simulink model "atrias_system"  (R2014b)
settings: Solver=FixedStepDiscrete  StartTime=0.0  StopTime=inf  FixedStep=sample_time  RelTol=1e-3
values from neighbouring files (symbols this model uses):
  MEDULLA_TIMER_FREQ = 32e6    (= 32000000)    [Encoder.m]
  sample_time = 0.001    [Encoder.m]
undefined symbols (not defined in the file or in its folder): A_lpf_velocity, B1_lpf_velocity, B2_lpf_velocity, BOOM_MAX_ENCODER_TICKS, BOOM_PITCH_CAL_VALUE_RAD, BOOM_PITCH_CAL_VALUE_TICKS, BOOM_PITCH_ENCODER_RAD_PER_TICK, BOOM_ROLL_CAL_VALUE_RAD, BOOM_ROLL_CAL_VALUE_TICKS, BOOM_ROLL_ENCODER_RAD_PER_TICK, BOOM_YAW_ENCODER_RAD_PER_TICK, fcut_smooth, fcut_unwrap, gui_disable_cmd, gui_enable_cmd, gui_estop_cmd, gui_reset_cmd, HIP_ABS_MAX_ENCODER_TICKS, HIP_CURRENT_LIMIT, HIP_INC_MAX_ENCODER_TICKS, HIP_MOTOR_CONSTANT, HIP_MTR_GEAR_RATIO, HIP_MTR_MAX_TORQUE, isOsuRobot, LEFT_HIP_ABS_ENCODER_RAD_PER_TICK, LEFT_HIP_CALIB_POS, LEFT_HIP_CALIB_VAL, LEFT_HIP_INC_ENCODER_RAD_PER_TICK, LEFT_MOTOR_HIP_DIRECTION, LEG1_LEG_A_CALIB_VAL, LEG1_LEG_A_RAD_PER_CNT, LEG1_LEG_B_CALIB_VAL, LEG1_LEG_B_RAD_PER_CNT, LEG1_MOTOR_A_DIRECTION, LEG1_MOTOR_B_DIRECTION, LEG1_TRAN_A_CALIB_VAL, LEG1_TRAN_A_RAD_PER_CNT, LEG1_TRAN_B_CALIB_VAL, LEG1_TRAN_B_RAD_PER_CNT, LEG2_LEG_A_CALIB_VAL, LEG2_LEG_A_RAD_PER_CNT, LEG2_LEG_B_CALIB_VAL, LEG2_LEG_B_RAD_PER_CNT, LEG2_MOTOR_A_DIRECTION, LEG2_MOTOR_B_DIRECTION, LEG2_TRAN_A_CALIB_VAL, LEG2_TRAN_A_RAD_PER_CNT, LEG2_TRAN_B_CALIB_VAL, LEG2_TRAN_B_RAD_PER_CNT, LEG_A_CALIB_LOC, LEG_B_CALIB_LOC, LEG_CURRENT_LIMIT, LEG_INC_ENCODER_RAD_PER_TICK, LEG_MOTOR_CONSTANT, LEG_MTR_GEAR_RATIO, LEG_MTR_MAX_TORQUE, max_encoder_velocity, max_sensor_velocity, MEDULLA_ADC_MAX_VOLTS, MEDULLA_ADC_OFFSET_COUNTS ... (+17)
libraries: xpcethercatlib x201, simulink x53, slrtlib x2
(part 1 of 4)
settings Model: xpc_rtwmakecfg_data=_xpcethercatlib_  SimulationMode=external  BufferReuse=off  Creator=wmartin  LastModifiedBy=drl
settings SolverCC: EnableConcurrentExecution=on
settings DataIOCC: MaxDataPoints=1000000000  SaveFormat=StructureWithTime  SaveOutput=off  SaveTime=off
settings OptimizationCC: BlockReduction=off  OptimizeBlockIOStorage=off  BufferReuse=off  GlobalBufferReuse=off  ExpressionFolding=off  ExpressionDepthLimit=2147483647  LocalBlockOutputs=off  SimCompilerOptimization=On
settings DebuggingCC: UnderspecifiedInitializationDetection=Classic  MergeDetectMultiDrivingBlocksExec=none  StateNameClashWarn=warning
settings HardwareCC: ProdIntDivRoundTo=Zero  ProdEndianess=LittleEndian  ProdLongLongMode=on  ProdHWDeviceType=Generic->32-bit x86 compatible
settings ModelReferenceCC: EnableParallelModelReferenceBuilds=on  ModelReferenceNumInstancesAllowed=Single  ModelReferenceMinAlgLoopOccurrences=on
settings RTWCC: SystemTargetFile=slrt.tlc  TemplateMakefile=slrt_default_tmf  Description=Simulink Real-Time  RTWVerbose=off  ProcessScript=slrt_make_rtw_hook  RTWCompilerOptimization=On
settings CodeAppCC: MaxIdLength=256
settings SimulinkRealTimeCC: GeneratePreprocessorConditionals=Disable all  EnableShiftOperators=on  RL32LogBufSizeModifier=100000000

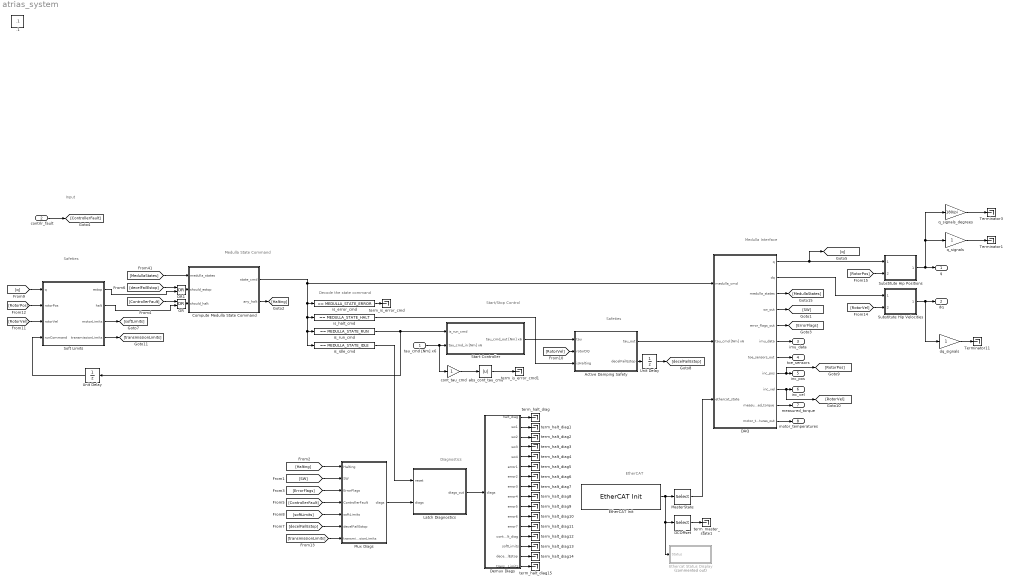
== system atrias_system ==
  note: Decode the state command
  note: Medulla Interface
  note: Medulla State Command
  note: Diagnostics
  note: EtherCAT
  note: Start/Stop Control
  note: Input
  note: Safeties
  note: Safeties
  tau_cmd [Nm] x6 : Inport
  contrlr_fault : Inport  Port=2  OutDataTypeStr=boolean
  Active Damping Safety : MATLAB Function  TreatAsAtomicUnit=on
  Compute Medulla State Command : MATLAB Function  TreatAsAtomicUnit=on
  DAQ : Subsystem
  DCOffset : Selector  InputPortWidth=6  Indices=[4]
  Demux Diags : MATLAB Function  TreatAsAtomicUnit=on
  EtherCAT Init : xpcethercatlib/EtherCAT Init   Priority=0  config_file=8medullas4elmos_eni.xml  device_id=0  pci_bus=2  pci_slot=0  enaDebug=off  enaDC=on  errLink=off  masterDbg=off  stateChgDbg=off  baseClock=off  masterCfg=off  logFile='E:\dbglog.txt'  sample_time=0.001000
  Ethercat Status Display : Subsystem  Commented=on
  Latch Diagnostics : MATLAB Function  TreatAsAtomicUnit=on
  MasterState : Selector  InputPortWidth=6  Indices=[2]
  Mux Diags : MATLAB Function  TreatAsAtomicUnit=on
  OR : Logic  Operator=OR  AllPortsSameDT=off  OutDataTypeStr=boolean
  OR1 : Logic  Operator=OR  AllPortsSameDT=off  OutDataTypeStr=boolean
  Soft Limits : MATLAB Function  TreatAsAtomicUnit=on
  Start Controller : Subsystem
  Substitute Hip Positions : Subsystem
  Substitute Hip Velocities : Subsystem
  Terminator1 : Terminator
  Terminator11 : Terminator
  Terminator3 : Terminator
  Unit Delay : UnitDelay  SampleTime=-1
  "Unit Delay " : UnitDelay  SampleTime=-1
  abs_cont_tau_cmd : Abs
  cont_tau_cmd : Gain
  dq_signals : Gain
  is_error_cmd : simulink/Logic and Bit Operations/Compare To Constant  relop===  const=MEDULLA_STATE_ERROR  OutDataTypeStr=boolean
  is_halt_cmd : simulink/Logic and Bit Operations/Compare To Constant  relop===  const=MEDULLA_STATE_HALT  OutDataTypeStr=boolean
  is_idle_cmd : simulink/Logic and Bit Operations/Compare To Constant  relop===  const=MEDULLA_STATE_IDLE  OutDataTypeStr=boolean
  is_run_cmd : simulink/Logic and Bit Operations/Compare To Constant  relop===  const=MEDULLA_STATE_RUN  OutDataTypeStr=boolean
  q_signals : Gain
  q_signals_degrees : Gain  Gain=180/pi
  term_halt_diag{,1..15} (16 alike) : Terminator
  term_is_error_cmd : Terminator
  term_is_error_cmd1 : Terminator
  term_master_state1 : Terminator
  q : Outport
  dq : Outport  Port=2
  imu_data : Outport  Port=3
  toe_sensors : Outport  Port=4
  inc_pos : Outport  Port=5
  inc_vel : Outport  Port=6
  measured_torque : Outport  Port=7
  motor_temperatures : Outport  Port=8
  .1 : Constant  IOType=siggen  Value=.1
  wires:
  MasterState/1 -> DAQ/3(ethercat_state)
  [MedullaStates] -> Compute Medulla State Command/1(medulla_states)
  Compute Medulla State Command/2(any_halt) -> [Halting]
  Latch Diagnostics/1(diags_out) -> Demux Diags/1(diags)
  is_halt_cmd/1 -> Active Damping Safety/3(isHalting)
  is_error_cmd/1 -> term_is_error_cmd/1
  tau_cmd [Nm] x6/1 -> cont_tau_cmd/1, Start Controller/2(tau_cmd_in [Nm] x6)
  Start Controller/1(tau_cmd_out [Nm] x6) -> Active Damping Safety/1(tau)
  is_idle_cmd/1 -> Latch Diagnostics/1(reset)
  DAQ/4(sw_out) -> [SW]
  Mux Diags/1(diags) -> Latch Diagnostics/2(diags)
  [Halting] -> Mux Diags/1(Halting)
  [SW] -> Mux Diags/2(SW)
  Demux Diags/2(sw1) -> term_halt_diag1/1
  Demux Diags/5(sw4) -> term_halt_diag4/1
  Demux Diags/4(sw3) -> term_halt_diag3/1
  Demux Diags/3(sw2) -> term_halt_diag2/1
  DAQ/5(error_flags_out) -> [ErrorFlags]
  [ErrorFlags] -> Mux Diags/3(ErrorFlags)
  Demux Diags/1(halt_diag) -> term_halt_diag/1
  Demux Diags/12(error7) -> term_halt_diag11/1
  Demux Diags/11(error6) -> term_halt_diag10/1
  Demux Diags/10(error5) -> term_halt_diag9/1
  Demux Diags/9(error4) -> term_halt_diag8/1
  Demux Diags/8(error3) -> term_halt_diag7/1
  Demux Diags/7(error2) -> term_halt_diag6/1
  Demux Diags/6(error1) -> term_halt_diag5/1
  abs_cont_tau_cmd/1 -> term_is_error_cmd1/1
  DAQ/6(imu_data) -> imu_data/1
  [ControllerFault] -> Mux Diags/4(ControllerFault)
  Demux Diags/13(contrlr_fault_diag) -> term_halt_diag12/1
  [RotorPos] -> Soft Limits/2(rotorPos)
  [RotorVel] -> Soft Limits/3(rotorVel)
  EtherCAT Init/1 -> DCOffset/1, Ethercat Status Display/1(Status), MasterState/1
  Compute Medulla State Command/1(state_cmd) -> is_idle_cmd/1, is_run_cmd/1, is_halt_cmd/1, is_error_cmd/1, DAQ/1(medulla_cmd)
  cont_tau_cmd/1 -> abs_cont_tau_cmd/1
  DAQ/7(toe_sensors_out) -> toe_sensors/1
  contrlr_fault/1 -> [ControllerFault]
  [softLimits] -> Mux Diags/5(softLimits)
  Demux Diags/14(softLimits) -> term_halt_diag13/1
  Soft Limits/3(motorLimits) -> [softLimits]
  is_run_cmd/1 -> Unit Delay/1, Start Controller/1(is_run_cmd)
  Active Damping Safety/1(tau_out) -> DAQ/2(tau_cmd [Nm] x6)
  [RotorVel] -> Active Damping Safety/2(rotorDQ)
  DCOffset/1 -> term_master_state1/1
  [q] -> Soft Limits/1(q)
  [decelFailEstop] -> Mux Diags/6(decelFailEstop)
  Demux Diags/15(decelFailEstop) -> term_halt_diag14/1
  DAQ/3(medulla_states) -> [MedullaStates]
  Active Damping Safety/2(decelFailEstop) -> "Unit Delay "/1
  "Unit Delay "/1 -> [decelFailEstop]
  DAQ/10(measured_torque) -> measured_torque/1
  DAQ/9(inc_vel) -> [RotorVel], inc_vel/1
  DAQ/8(inc_pos) -> [RotorPos], inc_pos/1
  [ControllerFault] -> OR/1
  Soft Limits/2(halt) -> OR/2
  OR/1 -> Compute Medulla State Command/3(should_halt)
  Unit Delay/1 -> Soft Limits/4(runCommand)
  [decelFailEstop] -> OR1/1
  OR1/1 -> Compute Medulla State Command/2(should_estop)
  Soft Limits/1(estop) -> OR1/2
  Soft Limits/4(transmissionLimits) -> [transmissionLimits]
  [transmissionLimits] -> Mux Diags/7(transmissionLimits)
  Demux Diags/16(transmissionLimits) -> term_halt_diag15/1
  DAQ/11(motor_temperatures_out) -> motor_temperatures/1
  [RotorVel] -> Substitute Hip Velocities/2(Incremental)
  DAQ/2(dq) -> Substitute Hip Velocities/1(Absolute)
  DAQ/1(q) -> Substitute Hip Positions/1(Absolute), [q]
  [RotorPos] -> Substitute Hip Positions/2(Incremental)
  q_signals/1 -> Terminator1/1
  q_signals_degrees/1 -> Terminator3/1
  Substitute Hip Positions/1(Substituted) -> q_signals_degrees/1, q_signals/1, q/1
  Substitute Hip Velocities/1(Substituted) -> dq_signals/1, dq/1
  dq_signals/1 -> Terminator11/1

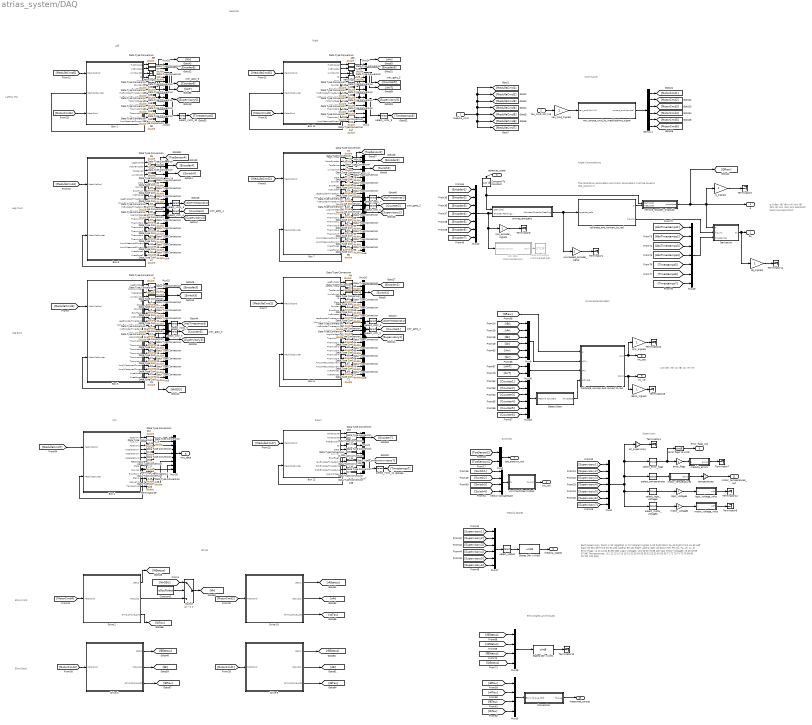
== system atrias_system/DAQ ==
  note: Left
  note: The calibration parameters and motor parameters
      | must be saved in daq_params.m
  note: Right
  note: Lateral Hip
  note: Leg Back
  note: Leg Front
  note: Boom
  note: Medullas
  note: Angle Computations
  note: Commands
  note: Switches
  note: Supervisory
  note: Each Supervisory block is 20 (sagittal) or 12 (lateral) signals
      | 1-20      Right Back
      | 21-40     Right Front
      | 41-60     Left Back
      | 61-80     Left Front
      | 81-92     Left Lateral
      | 93-104    Right Lateral
      | 105-112   Boom
      |
      | BR, FR, BL, FL, LR, LL, B
      | Error Flags: [4 24 44 64 84 96 108]
      | Logic Voltages: [10 30 50 70 88 100 112]
      | Motor Voltages: [9 29 49 69 87 99]
      | Temperatures: [11 12 13 14 15 16 31 32 33 34 35 36 51 52 53 54 55 56 71 72 73 74 75 76 89 90 91 101 102 103]
  note: q Order:
      |
      | rBl
      | rBm
      | rAl
      | rAm
      |
      | lBl
      | lBm
      | lAl
      | lAm
      |
      | rHm
      | lHm
      |
      | boomRoll
      | boomYaw
      | boomPitch
  note: Medulla States
  note: IMU
  note: Elmos
  note: Elmo Front
  note: Elmo Back
  note: Elmo States and Torques
  note: Incremental Encoders
  note: q Order:
      |
      | rBr
      | rAr
      | lBr
      | lAr
      |
      | rHr
      | lHr
  medulla_cmd : Inport
  tau_cmd [Nm] x6 : Inport  Port=2  OutDataTypeStr=double  PortDimensions=6  SampleTime=0
  ethercat_state : Inport  Port=3
  Box 1 : Subsystem
  Box 11 : Subsystem
  Box 12 : Subsystem
  Box 4 : Subsystem
  Box 5 : Subsystem
  Box 6 : Subsystem
  Box 7 : Subsystem
  Box 8 : Subsystem
  "Calibrate, unwrap, and convert to rad" : MATLAB Function  TreatAsAtomicUnit=on
  Compare To Constant : simulink/Logic and Bit Operations/Compare To Constant  relop===  const=8  OutDataTypeStr=boolean
  Constant1 : Constant  Value=isOsuRobot  OutDataTypeStr=Inherit: Inherit via back propagation
  Conversion : Subsystem
  Data Type Conversion{1..120,127..147,149..151} (144 alike) : DataTypeConversion  OutDataTypeStr=double
  Demux1 : Demux  Outputs=6
  Derivative : Subsystem
  Detect Data : Subsystem
  Drive 10 : Subsystem
  Drive 2 : Subsystem
  Drive 3 : Subsystem
  Drive 9 : Subsystem
  Error flags to uint8 : DataTypeConversion  OutDataTypeStr=uint8
  Fail Safe : Subsystem  Commented=on
  Limit Switches to Bool : MATLAB Function  TreatAsAtomicUnit=on
  Mux1 : Mux  Inputs=12
  Mux10 : Mux  Inputs=12
  Mux{2,11..16,18..20,24,30} (12 alike) : Mux  Inputs=2
  Mux17 : Mux  Inputs=6
  Mux21 : Mux  Inputs=3
  Mux22 : Mux  Inputs=7
  Mux23 : Mux  Inputs=6
  Mux25 : Mux
  Mux26 : Mux  Inputs=9
  Mux28 : Mux
  Mux29 : Mux  Inputs=7
  Mux{3..6} (4 alike) : Mux  Inputs=20
  Mux7 : Mux  Inputs=8
  Mux8 : Mux  Inputs=7
  Mux9 : Mux  Inputs=6
  States Dbl->Uint1 : DataTypeConversion  OutDataTypeStr=uint8
  States Dbl->Uint8 : DataTypeConversion  OutDataTypeStr=uint8
  Stop Simulation : Stop  Commented=on
  Switch : Switch  Criteria=u2 ~= 0  Threshold=max_sensor_velocity*sample_time
      settings: AttributesFormatString=%<Criteria>
  Terminator{1,3..4,6..14,19,22..25} (17 alike) : Terminator
  Vector Concatenate : Concatenate  NumInputs=4
  all_supervisory : Gain
  calibrate_and_convert_to_rad : Subsystem
  dq_signals : Gain
  dqinc_signals : Gain
  error_flags : Gain
  logic_voltage_volts : MATLAB Function  TreatAsAtomicUnit=on
  logic_voltages : Gain
  medulla_errors : MATLAB Function  TreatAsAtomicUnit=on
  motor_temperatures : MATLAB Function  TreatAsAtomicUnit=on
  motor_voltage_volts : MATLAB Function  TreatAsAtomicUnit=on
  motor_voltages : Gain
  mtr_torque_cmd_to_medulla/elmo_signal : Subsystem
  q_signals : Gain
  qinc_signals : Gain
  raw_encoder_signals : Gain
  remove_encoder_dropouts : Subsystem
  select_cntr_{1..4} (4 alike) : Selector  InputPortWidth=20  Indices=3
  select_error_flags : Selector  InputPortWidth=112  Indices=[4 24 44 64 84 96 108]
  select_incts_10 : Selector  InputPortWidth=12  Indices=[6]
  select_incts_11 : Selector  InputPortWidth=8  Indices=[5 6 7]
  select_incts_{5..8} (4 alike) : Selector  InputPortWidth=20  Indices=[6 7]
  select_incts_9 : Selector  InputPortWidth=12  Indices=[6]
  select_logic_voltages : Selector  InputPortWidth=112  Indices=[10 30 50 70 88 100 112]
  select_motor_voltages : Selector  InputPortWidth=112  Indices=[9 29 49 69 87 99]
  select_states : Selector  InputPortWidth=104  Indices=[2 22 42 62 82 94]
  select_temperatures : Selector  InputPortWidth=112  Indices=[11 12 13 14 15 16 31 32 33 34 35 36 51 52 53 54 55 56 71 72 73 74 75 76 89 90 91 101 102 103]
  tau_cmd_signals : Gain
  temperatures : Gain
  unwrap_encoders : Subsystem
  unwrapped_encoder_signal : Gain
  q : Outport  OutDataTypeStr=double  PortDimensions=13  SampleTime=[0.001,0]
  dq : Outport  Port=2  OutDataTypeStr=double  PortDimensions=13  SampleTime=[0.001,0]
  medulla_states : Outport  Port=3  OutDataTypeStr=uint8
  sw_out : Outport  Port=4
  error_flags_out : Outport  Port=5  OutDataTypeStr=uint8
  imu_data : Outport  Port=6
  toe_sensors_out : Outport  Port=7
  inc_pos : Outport  Port=8
  inc_vel : Outport  Port=9
  measured_torque : Outport  Port=10
  motor_temperatures_out : Outport  Port=11
  wires:
  Box 12/11(LogicVoltage) -> Data Type Conversion136/1
  Box 12/10(PitchEncoderTimestamp) -> Data Type Conversion137/1
  Box 12/9(RollEncoderTimestamp) -> Data Type Conversion127/1
  Box 12/8(YawEncoderTimestamp) -> Data Type Conversion129/1
  Box 12/7(ErrorFlags) -> Data Type Conversion130/1
  Box 12/5(State) -> Data Type Conversion134/1
  Box 12/4(ID) -> Data Type Conversion135/1
  Box 12/3(PitchEncoder) -> Data Type Conversion131/1
  Box 12/2(YawEncoder) -> Data Type Conversion132/1
  Box 12/1(RollEncoder) -> Data Type Conversion133/1
  Data Type Conversion133/1 -> Mux21/1
  Data Type Conversion132/1 -> Mux21/2
  Data Type Conversion131/1 -> Mux21/3
  Data Type Conversion135/1 -> Mux7/1
  Data Type Conversion134/1 -> Mux7/2
  Data Type Conversion128/1 -> Mux7/3
  Data Type Conversion130/1 -> Mux7/4
  Data Type Conversion129/1 -> Mux7/5
  Data Type Conversion127/1 -> Mux7/6
  Data Type Conversion137/1 -> Mux7/7
  Data Type Conversion136/1 -> Mux7/8
  Data Type Conversion98/1 -> Mux18/1
  Data Type Conversion97/1 -> [lHr], Mux18/2
  Data Type Conversion110/1 -> Mux10/1
  Data Type Conversion105/1 -> Mux10/2
  Data Type Conversion107/1 -> [Counter6], Mux10/3
  Data Type Conversion106/1 -> Mux10/4
  Data Type Conversion109/1 -> Mux10/5
  Data Type Conversion101/1 -> Mux10/7
  Data Type Conversion103/1 -> Mux10/8
  Data Type Conversion102/1 -> Mux10/9
  Data Type Conversion100/1 -> Mux10/10
  Data Type Conversion99/1 -> Mux10/11
  mtr_torque_cmd_to_medulla/elmo_signal/1(current_cmd [counts]) -> Demux1/1
  Data Type Conversion50/1 -> Mux16/2
  Data Type Conversion49/1 -> Mux16/1
  Data Type Conversion48/1 -> Mux4/20
  Data Type Conversion47/1 -> Mux4/19
  Data Type Conversion46/1 -> Mux4/18
  Data Type Conversion45/1 -> Mux4/17
  Data Type Conversion44/1 -> Mux4/16
  Data Type Conversion43/1 -> Mux4/15
  Data Type Conversion42/1 -> Mux4/14
  Data Type Conversion41/1 -> Mux4/13
  Data Type Conversion40/1 -> Mux4/12
  Data Type Conversion39/1 -> Mux4/11
  Data Type Conversion38/1 -> Mux4/10
  Data Type Conversion37/1 -> Mux4/9
  Data Type Conversion36/1 -> Mux4/8
  Data Type Conversion35/1 -> Mux4/7
  Data Type Conversion34/1 -> Mux4/6
  Data Type Conversion33/1 -> Mux4/5
  Data Type Conversion32/1 -> Mux4/4
  Data Type Conversion31/1 -> Mux4/3
  Data Type Conversion30/1 -> Mux4/2
  Data Type Conversion29/1 -> Mux4/1
  Data Type Conversion27/1 -> Mux14/1, [ToeSensor4]
  Data Type Conversion26/1 -> Mux20/2
  Data Type Conversion25/1 -> Mux20/1
  Data Type Conversion24/1 -> Mux3/20
  Data Type Conversion23/1 -> Mux3/19
  Data Type Conversion22/1 -> Mux3/18
  Data Type Conversion21/1 -> Mux3/17
  Data Type Conversion20/1 -> Mux3/16
  Data Type Conversion19/1 -> Mux3/15
  Data Type Conversion18/1 -> Mux3/14
  Data Type Conversion17/1 -> Mux3/13
  Data Type Conversion16/1 -> Mux3/12
  Data Type Conversion15/1 -> Mux3/11
  Data Type Conversion14/1 -> Mux3/10
  Data Type Conversion13/1 -> Mux3/9
  Data Type Conversion12/1 -> Mux3/8
  Data Type Conversion11/1 -> Mux3/7
  Data Type Conversion10/1 -> Mux3/6
  Data Type Conversion9/1 -> [lArOSU], Mux3/5
  Data Type Conversion8/1 -> Mux3/4
  Data Type Conversion7/1 -> Mux3/3
  Data Type Conversion6/1 -> Mux3/2
  Data Type Conversion5/1 -> Mux3/1
  Data Type Conversion2/1 -> Mux13/1
  Data Type Conversion1/1 -> Mux15/2
  Data Type Conversion3/1 -> Mux15/1
  tau_cmd [Nm] x6/1 -> tau_cmd_signals/1
  Data Type Conversion138/1 -> Mux10/12
  Data Type Conversion96/1 -> Mux6/20
  Data Type Conversion95/1 -> Mux6/19
  Data Type Conversion94/1 -> Mux6/18
  Data Type Conversion93/1 -> Mux6/17
  Data Type Conversion92/1 -> Mux6/16
  Data Type Conversion91/1 -> Mux6/15
  Data Type Conversion90/1 -> Mux6/14
  Data Type Conversion89/1 -> Mux6/13
  Data Type Conversion88/1 -> Mux6/12
  Data Type Conversion87/1 -> Mux6/11
  Data Type Conversion86/1 -> Mux6/10
  Data Type Conversion85/1 -> Mux6/9
  Data Type Conversion84/1 -> Mux6/8
  Data Type Conversion83/1 -> Mux6/7
  Data Type Conversion82/1 -> Mux6/6
  Data Type Conversion81/1 -> Mux6/5
  Data Type Conversion80/1 -> Mux6/4
  Data Type Conversion79/1 -> Mux6/3
  Data Type Conversion78/1 -> Mux6/2
  Data Type Conversion77/1 -> Mux6/1
  Data Type Conversion75/1 -> Mux11/1, [ToeSensor2]
  Data Type Conversion74/1 -> Mux19/2
  Data Type Conversion73/1 -> Mux19/1
  Data Type Conversion72/1 -> Mux5/20
  Data Type Conversion71/1 -> Mux5/19
  Data Type Conversion70/1 -> Mux5/18
  Data Type Conversion69/1 -> Mux5/17
  Data Type Conversion68/1 -> Mux5/16
  Data Type Conversion67/1 -> Mux5/15
  Data Type Conversion66/1 -> Mux5/14
  Data Type Conversion65/1 -> Mux5/13
  Data Type Conversion64/1 -> Mux5/12
  Data Type Conversion63/1 -> Mux5/11
  Data Type Conversion62/1 -> Mux5/10
  Data Type Conversion61/1 -> Mux5/9
  Data Type Conversion60/1 -> Mux5/8
  Data Type Conversion59/1 -> Mux5/7
  Data Type Conversion58/1 -> Mux5/6
  Data Type Conversion57/1 -> Mux5/5
  Data Type Conversion56/1 -> Mux5/4
  Data Type Conversion55/1 -> Mux5/3
  Data Type Conversion54/1 -> Mux5/2
  Data Type Conversion53/1 -> Mux5/1
  Data Type Conversion51/1 -> Mux12/1
  Box 12/6(Counter) -> Box 12/2(MedullaCounter), Data Type Conversion128/1
  [MedullaCmd7] -> Box 12/1(MedullaCmd)
  Derivative/1(dq) -> dq_signals/1, dq/1
  Demux1/1 -> [MotorCmd1]
  Demux1/2 -> [MotorCmd2]
  Demux1/3 -> [MotorCmd3]
  Demux1/4 -> [MotorCmd4]
  Demux1/5 -> [MotorCmd5]
  Demux1/6 -> [MotorCmd6]
  Mux3/1 -> select_incts_5/1, select_cntr_3/1, [Supervisory3]
  Mux4/1 -> [Supervisory4], select_incts_6/1, select_cntr_4/1
  Mux5/1 -> [Supervisory1], select_incts_8/1, select_cntr_1/1
  Mux6/1 -> select_incts_7/1, select_cntr_2/1, [Supervisory2]
  [Supervisory1] -> Mux8/1
  [Supervisory2] -> Mux8/2
  [Supervisory3] -> Mux8/3
  [Supervisory4] -> Mux8/4
  [Supervisory5] -> Mux8/5
  [Supervisory6] -> Mux8/6
  [Supervisory7] -> Mux8/7
  Mux15/1 -> [Encoder3]
  Mux16/1 -> [Encoder1]
  Mux18/1 -> [Encoder6]
  Mux19/1 -> [Encoder2]
  Mux20/1 -> [Encoder4]
  Mux21/1 -> [Encoder7]
  [Encoder7] -> Mux22/7
  [Encoder6] -> Mux22/6
  [Encoder5] -> Mux22/5
  [Encoder4] -> Mux22/4
  [Encoder3] -> Mux22/3
  [Encoder2] -> Mux22/2
  [Encoder1] -> Mux22/1
  Data Type Conversion150/1 -> Mux24/1
  Data Type Conversion149/1 -> [rHr], Mux24/2
  Data Type Conversion146/1 -> Mux1/1
  Data Type Conversion141/1 -> Mux1/2
  Data Type Conversion143/1 -> [Counter5], Mux1/3
  Data Type Conversion142/1 -> Mux1/4
  Data Type Conversion145/1 -> Mux1/5
  Data Type Conversion144/1 -> [rHrT], Mux1/6
  Data Type Conversion111/1 -> Mux1/7
  Data Type Conversion140/1 -> Mux1/8
  Data Type Conversion139/1 -> Mux1/9
  Data Type Conversion104/1 -> Mux1/10
  Data Type Conversion151/1 -> Mux1/11
  Data Type Conversion147/1 -> Mux1/12
  Mux24/1 -> [Encoder5]
  tau_cmd_signals/1 -> mtr_torque_cmd_to_medulla/elmo_signal/1(tau_cmd [Nm] x6)
  Mux8/1 -> select_temperatures/1, select_error_flags/1, all_supervisory/1, select_motor_voltages/1, select_logic_voltages/1
  select_error_flags/1 -> error_flags/1, Error flags to uint8/1
  select_logic_voltages/1 -> logic_voltages/1
  select_motor_voltages/1 -> motor_voltages/1
  calibrate_and_convert_to_rad/1(q) -> remove_encoder_dropouts/2(measured)
  all_supervisory/1 -> Terminator4/1
  motor_voltage_volts/1(volt) -> Terminator6/1
  medulla_errors/1(errors) -> Terminator7/1
  logic_voltage_volts/1(volt) -> Terminator12/1
  medulla_cmd/1 -> [MedullaCmd3], [MedullaCmd2], [MedullaCmd1], [MedullaCmd4], [MedullaCmd6], [MedullaCmd7], [MedullaCmd5]
  [Supervisory1] -> Mux17/1
  [Supervisory2] -> Mux17/2
  [Supervisory3] -> Mux17/3
  [Supervisory4] -> Mux17/4
  [Supervisory5] -> Mux17/5
  [Supervisory6] -> Mux17/6
  Mux17/1 -> select_states/1
  select_states/1 -> States Dbl->Uint8/1
  States Dbl->Uint8/1 -> medulla_states/1
  [Switch1] -> Vector Concatenate/1
  [Switch2] -> Vector Concatenate/2
  [Switch3] -> Vector Concatenate/3
  [Switch4] -> Vector Concatenate/4
  Vector Concatenate/1 -> Limit Switches to Bool/1(sw)
  Limit Switches to Bool/1(sw_out) -> sw_out/1
  Error flags to uint8/1 -> error_flags_out/1
  select_cntr_1/1 -> [Counter1]
  select_cntr_2/1 -> [Counter2]
  select_cntr_3/1 -> [Counter3]
  select_cntr_4/1 -> [Counter4]
  Box 4/3(RotationZ) -> Data Type Conversion114/1
  Box 4/4(AccelerationX) -> Data Type Conversion115/1
  Box 4/5(AccelerationY) -> Data Type Conversion116/1
  Box 4/6(AccelerationZ) -> Data Type Conversion117/1
  Data Type Conversion112/1 -> Mux26/1
  Data Type Conversion113/1 -> Mux26/2
  Data Type Conversion114/1 -> Mux26/3
  Box 4/7(ID) -> Terminator9/1
  Box 4/8(State) -> Terminator13/1
  Box 4/13(Temperature) -> Terminator19/1
  Box 4/10(ErrorFlags) -> Terminator14/1
  Data Type Conversion117/1 -> Mux26/6
  Data Type Conversion116/1 -> Mux26/5
  Data Type Conversion115/1 -> Mux26/4
  Mux26/1 -> imu_data/1
  [MedullaCmd7] -> Box 4/1(MedullaCmd)
  Box 4/9(Counter) -> Data Type Conversion119/1, Box 4/2(MedullaCounter)
  raw_encoder_signals/1 -> Terminator8/1
  select_incts_5/1 -> [AbsTimestamps3]
  select_incts_6/1 -> [AbsTimestamps4]
  select_incts_7/1 -> [AbsTimestamps2]
  select_incts_8/1 -> [AbsTimestamps1]
  calibrate_and_convert_to_rad/2(hip_inc) -> Derivative/2(hip_inc)
  [rBStatus] -> Mux28/1
  States Dbl->Uint1/1 -> Terminator10/1
  Mux28/1 -> States Dbl->Uint1/1
  [rAStatus] -> Mux28/2
  [lBStatus] -> Mux28/3
  [lAStatus] -> Mux28/4
  [AbsTimestamps1] -> Mux29/1
  [AbsTimestamps2] -> Mux29/2
  [AbsTimestamps3] -> Mux29/3
  [AbsTimestamps4] -> Mux29/4
  select_incts_9/1 -> [Timestamps5]
  Mux1/1 -> select_incts_9/1, [Supervisory5]
  select_incts_10/1 -> [Timestamps6]
  Mux10/1 -> select_incts_10/1, [Supervisory6]
  [Timestamps5] -> Mux29/5
  [Timestamps6] -> Mux29/6
  Mux29/1 -> Derivative/3(timestamps)
  select_incts_11/1 -> [Timestamps7]
  Mux7/1 -> select_incts_11/1, [Supervisory7]
  [Timestamps7] -> Mux29/7
  Box 1/1(HipEncoder) -> Data Type Conversion98/1
  Box 1/2(IncEncoder) -> Data Type Conversion97/1
  Box 1/4(ID) -> Data Type Conversion110/1
  Box 1/5(State) -> Data Type Conversion105/1
  Box 1/7(ErrorFlags) -> Data Type Conversion106/1
  Box 1/8(HipEncoderTimestamp) -> Data Type Conversion109/1
  Box 1/9(IncEncoderTimestamp) -> Data Type Conversion108/1
  Box 1/10(MotorVoltage) -> Data Type Conversion101/1
  Box 1/11(LogicVoltage) -> Data Type Conversion103/1
  Box 1/12(Thermistor0) -> Data Type Conversion102/1
  Box 1/13(Thermistor1) -> Data Type Conversion100/1
  Box 1/14(Thermistor2) -> Data Type Conversion99/1
  Box 1/15(AmpMeasuredCurrent) -> Data Type Conversion138/1
  [MedullaCmd6] -> Box 1/1(MedullaCmd)
  Box 1/6(Counter) -> Box 1/2(MedullaCounter), Data Type Conversion107/1
  [MotorCmd6] -> Box 1/3(MotorCmd)
  [MedullaCmd5] -> Box 11/1(MedullaCmd)
  Box 11/6(Counter) -> Data Type Conversion143/1, Box 11/2(MedullaCounter)
  [MotorCmd5] -> Box 11/3(MotorCmd)
  Box 11/1(HipEncoder) -> Data Type Conversion150/1
  Box 11/2(IncEncoder) -> Data Type Conversion149/1
  Box 11/4(ID) -> Data Type Conversion146/1
  Box 11/5(State) -> Data Type Conversion141/1
  Box 11/7(ErrorFlags) -> Data Type Conversion142/1
  Box 11/8(HipEncoderTimestamp) -> Data Type Conversion145/1
  Box 11/9(IncEncoderTimestamp) -> Data Type Conversion144/1
  Box 11/10(MotorVoltage) -> Data Type Conversion111/1
  Box 11/11(LogicVoltage) -> Data Type Conversion140/1
  Box 11/12(Thermistor0) -> Data Type Conversion139/1
  Box 11/13(Thermistor1) -> Data Type Conversion104/1
  Box 11/14(Thermistor2) -> Data Type Conversion151/1
  Box 11/15(AmpMeasuredCurrent) -> Data Type Conversion147/1
  Box 5/1(LegEncoder) -> Data Type Conversion3/1
  Box 5/2(MotorEncoder) -> Data Type Conversion1/1
  Box 5/3(ToeSensor) -> Data Type Conversion2/1
  Box 5/4(LimitSwitch) -> Data Type Conversion4/1
  Box 5/5(ID) -> Data Type Conversion5/1
  Box 5/6(State) -> Data Type Conversion6/1
  Box 5/8(ErrorFlags) -> Data Type Conversion8/1
  Box 5/9(IncEncoder) -> Data Type Conversion9/1
  Box 5/10(LegEncoderTimestamp) -> Data Type Conversion10/1
  Box 5/11(MotorEncoderTimestamp) -> Data Type Conversion11/1
  Box 5/12(IncEncoderTimestamp) -> Data Type Conversion12/1
  Box 5/13(MotorVoltage) -> Data Type Conversion13/1
  Box 5/14(LogicVoltage) -> Data Type Conversion14/1
  Box 5/15(Thermistor0) -> Data Type Conversion15/1
  Box 5/16(Thermistor1) -> Data Type Conversion16/1
  Box 5/17(Thermistor2) -> Data Type Conversion17/1
  Box 5/18(Thermistor3) -> Data Type Conversion18/1
  Box 5/19(Thermistor4) -> Data Type Conversion19/1
  Box 5/20(Thermistor5) -> Data Type Conversion20/1
  Box 5/21(Amp1MeasuredCurrent) -> Data Type Conversion21/1
  Box 5/22(Amp2MeasuredCurrent) -> Data Type Conversion22/1
  Box 5/23(KneeForce1) -> Data Type Conversion23/1
  Box 5/24(KneeForce2) -> Data Type Conversion24/1
  [MedullaCmd3] -> Box 5/1(MedullaCmd)
  Box 5/7(Counter) -> Box 5/2(MedullaCounter), Data Type Conversion7/1
  [MotorCmd3] -> Drive 3/1(MotorCmd)
  Drive 3/1(status) -> [lBStatus]
  [MotorCmd1] -> Drive 9/1(MotorCmd)
  Drive 9/1(status) -> [rBStatus]
  [MotorCmd4] -> Drive 2/1(MotorCmd)
  Drive 2/1(status) -> [lAStatus]
  [ToeSensor4] -> Mux2/2
  [ToeSensor2] -> Mux2/1
  Mux2/1 -> toe_sensors_out/1
  Data Type Conversion76/1 -> Mux11/2
  Mux11/1 -> [Switch2]
  Data Type Conversion52/1 -> Mux12/2
  Mux12/1 -> [Switch1]
  Data Type Conversion4/1 -> Mux13/2
  Mux13/1 -> [Switch3]
  Data Type Conversion28/1 -> Mux14/2
  Mux14/1 -> [Switch4]
  error_flags/1 -> medulla_errors/1(u)
  logic_voltages/1 -> logic_voltage_volts/1(u)
  motor_voltages/1 -> motor_voltage_volts/1(u)
  Drive 3/2(rotor_tics) -> [lBr]
  Drive 9/2(rotor_tics) -> [rBr]
  [Counter1] -> Mux23/1
  [Counter2] -> Mux23/2
  [Counter3] -> Mux23/3
  [Counter4] -> Mux23/4
  [Counter5] -> Mux23/5
  [Counter6] -> Mux23/6
  [rBr] -> Mux9/1
  [rAr] -> Mux9/2
  [lBr] -> Mux9/3
  [lAr] -> Mux9/4
  Drive 9/3(elmo_torque_pdo) -> [rBTau]
  Drive 2/3(elmo_torque_pdo) -> [lATau]
  Drive 3/3(elmo_torque_pdo) -> [lBTau]
  [rBTau] -> Mux25/1
  [rATau] -> Mux25/2
  [lBTau] -> Mux25/3
  [lATau] -> Mux25/4
  Mux25/1 -> Conversion/1(Elmo Torque PDO)
  Conversion/1(Torque) -> measured_torque/1
  Mux9/1 -> "Calibrate, unwrap, and convert to rad"/2(qTic)
  "Calibrate, unwrap, and convert to rad"/1(qInc) -> inc_pos/1, qinc_signals/1
  "Calibrate, unwrap, and convert to rad"/2(dqInc) -> dqinc_signals/1, inc_vel/1
  [QRaw] -> "Calibrate, unwrap, and convert to rad"/1(q)
  Mux23/1 -> Detect Data/1(Medulla Counters)
  Detect Data/1(HaveData) -> "Calibrate, unwrap, and convert to rad"/4(activate)
  Data Type Conversion108/1 -> [lHrT], Mux10/6
  [lHr] -> Mux9/6
  [rHr] -> Mux9/5
  [lHrT] -> Mux30/2
  [rHrT] -> Mux30/1
  Mux30/1 -> "Calibrate, unwrap, and convert to rad"/3(tTic)
  qinc_signals/1 -> Terminator22/1
  dqinc_signals/1 -> Terminator23/1
  motor_temperatures/1(temp) -> temperatures/1
  select_temperatures/1 -> motor_temperatures/1(u)
  temperatures/1 -> motor_temperatures_out/1
  Box 1/3(LimitSwitch) -> Terminator24/1
  Box 11/3(LimitSwitch) -> Terminator25/1
  [MedullaCmd4] -> Box 6/1(MedullaCmd)
  Box 6/7(Counter) -> Box 6/2(MedullaCounter), Data Type Conversion31/1
  Box 6/1(LegEncoder) -> Data Type Conversion25/1
  Box 6/2(MotorEncoder) -> Data Type Conversion26/1
  Box 6/3(ToeSensor) -> Data Type Conversion27/1
  Box 6/4(LimitSwitch) -> Data Type Conversion28/1
  Box 6/5(ID) -> Data Type Conversion29/1
  Box 6/6(State) -> Data Type Conversion30/1
  Box 6/8(ErrorFlags) -> Data Type Conversion32/1
  Box 6/9(IncEncoder) -> Data Type Conversion33/1
  Box 6/10(LegEncoderTimestamp) -> Data Type Conversion34/1
  Box 6/11(MotorEncoderTimestamp) -> Data Type Conversion35/1
  Box 6/12(IncEncoderTimestamp) -> Data Type Conversion36/1
  Box 6/13(MotorVoltage) -> Data Type Conversion37/1
  Box 6/14(LogicVoltage) -> Data Type Conversion38/1
  Box 6/15(Thermistor0) -> Data Type Conversion39/1
  Box 6/16(Thermistor1) -> Data Type Conversion40/1
  Box 6/17(Thermistor2) -> Data Type Conversion41/1
  Box 6/18(Thermistor3) -> Data Type Conversion42/1
  Box 6/19(Thermistor4) -> Data Type Conversion43/1
  Box 6/20(Thermistor5) -> Data Type Conversion44/1
  Box 6/21(Amp1MeasuredCurrent) -> Data Type Conversion45/1
  Box 6/22(Amp2MeasuredCurrent) -> Data Type Conversion46/1
  Box 6/23(KneeForce1) -> Data Type Conversion47/1
  Box 6/24(KneeForce2) -> Data Type Conversion48/1
  [MedullaCmd2] -> Box 7/1(MedullaCmd)
  Box 7/7(Counter) -> Box 7/2(MedullaCounter), Data Type Conversion79/1
  Box 7/1(LegEncoder) -> Data Type Conversion73/1
  Box 7/2(MotorEncoder) -> Data Type Conversion74/1
  Box 7/3(ToeSensor) -> Data Type Conversion75/1
  Box 7/4(LimitSwitch) -> Data Type Conversion76/1
  Box 7/5(ID) -> Data Type Conversion77/1
  Box 7/6(State) -> Data Type Conversion78/1
  Box 7/8(ErrorFlags) -> Data Type Conversion80/1
  Box 7/9(IncEncoder) -> Data Type Conversion81/1
  Box 7/10(LegEncoderTimestamp) -> Data Type Conversion82/1
  Box 7/11(MotorEncoderTimestamp) -> Data Type Conversion83/1
  Box 7/12(IncEncoderTimestamp) -> Data Type Conversion84/1
  Box 7/13(MotorVoltage) -> Data Type Conversion85/1
  Box 7/14(LogicVoltage) -> Data Type Conversion86/1
  Box 7/15(Thermistor0) -> Data Type Conversion87/1
  Box 7/16(Thermistor1) -> Data Type Conversion88/1
  Box 7/17(Thermistor2) -> Data Type Conversion89/1
  Box 7/18(Thermistor3) -> Data Type Conversion90/1
  Box 7/19(Thermistor4) -> Data Type Conversion91/1
  Box 7/20(Thermistor5) -> Data Type Conversion92/1
  Box 7/21(Amp1MeasuredCurrent) -> Data Type Conversion93/1
  Box 7/22(Amp2MeasuredCurrent) -> Data Type Conversion94/1
  Box 7/23(KneeForce1) -> Data Type Conversion95/1
  Box 7/24(KneeForce2) -> Data Type Conversion96/1
  [MedullaCmd1] -> Box 8/1(MedullaCmd)
  Box 8/7(Counter) -> Box 8/2(MedullaCounter), Data Type Conversion55/1
  Box 8/1(LegEncoder) -> Data Type Conversion49/1
  Box 8/2(MotorEncoder) -> Data Type Conversion50/1
  Box 8/3(ToeSensor) -> Data Type Conversion51/1
  Box 8/4(LimitSwitch) -> Data Type Conversion52/1
  Box 8/5(ID) -> Data Type Conversion53/1
  Box 8/6(State) -> Data Type Conversion54/1
  Box 8/8(ErrorFlags) -> Data Type Conversion56/1
  Box 8/9(IncEncoder) -> Data Type Conversion57/1
  Box 8/10(LegEncoderTimestamp) -> Data Type Conversion58/1
  Box 8/11(MotorEncoderTimestamp) -> Data Type Conversion59/1
  Box 8/12(IncEncoderTimestamp) -> Data Type Conversion60/1
  Box 8/13(MotorVoltage) -> Data Type Conversion61/1
  Box 8/14(LogicVoltage) -> Data Type Conversion62/1
  Box 8/15(Thermistor0) -> Data Type Conversion63/1
  Box 8/16(Thermistor1) -> Data Type Conversion64/1
  Box 8/17(Thermistor2) -> Data Type Conversion65/1
  Box 8/18(Thermistor3) -> Data Type Conversion66/1
  Box 8/19(Thermistor4) -> Data Type Conversion67/1
  Box 8/20(Thermistor5) -> Data Type Conversion68/1
  Box 8/21(Amp1MeasuredCurrent) -> Data Type Conversion69/1
  Box 8/22(Amp2MeasuredCurrent) -> Data Type Conversion70/1
  Box 8/23(KneeForce1) -> Data Type Conversion71/1
  Box 8/24(KneeForce2) -> Data Type Conversion72/1
  [MotorCmd2] -> Drive 10/1(MotorCmd)
  Drive 10/1(status) -> [rAStatus]
  Drive 10/3(elmo_torque_pdo) -> [rATau]
  Box 4/12(Sequence) -> Data Type Conversion118/1
  Data Type Conversion118/1 -> Mux26/7
  Box 4/11(Status) -> Data Type Conversion120/1
  Box 4/1(RotationX) -> Data Type Conversion112/1
  Box 4/2(RotationY) -> Data Type Conversion113/1
  Data Type Conversion119/1 -> Mux26/9
  Data Type Conversion120/1 -> Mux26/8
  unwrapped_encoder_signal/1 -> Terminator1/1
  unwrap_encoders/1(Adjusted Encoder Readings) -> unwrapped_encoder_signal/1, calibrate_and_convert_to_rad/1(encoder_ticks)
  ethercat_state/1 -> Compare To Constant/1
  q_signals/1 -> Terminator3/1
  dq_signals/1 -> Terminator11/1
  Mux22/1 -> unwrap_encoders/2(Encoder Readings), Fail Safe/1(encoder signals), raw_encoder_signals/1
  Fail Safe/1(stop?) -> Stop Simulation/1
  remove_encoder_dropouts/1(smoothed) -> q/1, Derivative/1(q), q_signals/1, [QRaw]
  Compare To Constant/1 -> unwrap_encoders/1(Start [1/0]), remove_encoder_dropouts/1(Start [1/0])
  Constant1/1 -> Switch/2
  Drive 10/2(rotor_tics) -> [rAr]
  Switch/1 -> [lAr]
  [lArOSU] -> Switch/1
  Drive 2/2(rotor_tics) -> Switch/3

== system atrias_system/Ethercat Status Display ==
  Status : Inport
  Constant2 : Constant  Value=0  OutDataTypeStr=Inherit: Inherit via back propagation  SampleTime=-1
  Data Type Conversion{,1..6} (7 alike) : DataTypeConversion
  Demux : Demux  Outputs=6
  Discrete Filter2 : DiscreteFilter  Numerator="[0.001568334083281   0.001568334083281]"  Denominator="[1.000000000000000  -0.996863331833438]"  a0EqualsOne=on
  Mux2 : Mux  Inputs=3
  Mux3 : Mux  Inputs=6
  Scope 2 : slrtlib/Displays and Logging/Scope   scopeno=1  scopetype=Target  autostart=on  viewmode=Graphical rolling  formatstr='%f'  grid=on  ylimits=[0,0]  nosamples=10000  noprepostsamples=0  interleave=1  triggermode=FreeRun  triggersignal=1  trigsignalfromport=off  triggerlevel=0.0  triggerslope=Either  triggerscope=1  triggersample=0  filename=data.dat  mode=Lazy  writesize=512  autorestart=off  dynamicfilemode=off  maxwritefilesize=512*1024^2
  Scope 3 : slrtlib/Displays and Logging/Scope   scopeno=3  scopetype=Target  autostart=on  viewmode=Numerical  formatstr='%15.6f'  grid=on  ylimits=[0,0]  nosamples=100  noprepostsamples=0  interleave=1  triggermode=FreeRun  triggersignal=1  trigsignalfromport=off  triggerlevel=0.0  triggerslope=Either  triggerscope=1  triggersample=0  filename=data.dat  mode=Lazy  writesize=512  autorestart=off  dynamicfilemode=off  maxwritefilesize=512*1024^2
  wires:
  Status/1 -> Demux/1
  Demux/4 -> Discrete Filter2/1, Mux2/1
  Discrete Filter2/1 -> Data Type Conversion/1
  Mux2/1 -> Scope 2/1
  Constant2/1 -> Data Type Conversion4/1
  Data Type Conversion4/1 -> Mux2/3
  Mux3/1 -> Scope 3/1
  Data Type Conversion/1 -> Mux3/4, Mux2/2  "MasterRefToClockDiff"
  Data Type Conversion1/1 -> Mux3/1  "ErrVal"
  Data Type Conversion2/1 -> Mux3/2  "MasterState"
  Data Type Conversion3/1 -> Mux3/3  "DCErrVal"
  Data Type Conversion5/1 -> Mux3/5  "DCInitState"
  Data Type Conversion6/1 -> Mux3/6  "RefClockToSlaveDiff"
  Demux/1 -> Data Type Conversion1/1  "ErrVal"
  Demux/2 -> Data Type Conversion2/1  "MasterState"
  Demux/3 -> Data Type Conversion3/1  "DCErrVal"
  Demux/5 -> Data Type Conversion5/1  "DCInitState"
  Demux/6 -> Data Type Conversion6/1  "RefClockToSlaveDiff"

== system atrias_system/Start Controller ==
  note: For GUI
  note: Input Order:
      |
      | backR
      | frontR
      | latR
      | backL
      | frontL
      | latL
  is_run_cmd : Inport  OutDataTypeStr=boolean  PortDimensions=1
  tau_cmd_in [Nm] x6 : Inport  Port=2
  Current Time : Clock
  Enabled time : Sum  Inputs=-+
  Hold Start Time : Subsystem  TreatAsAtomicUnit=on
  Lateral Motor Saturation : Saturate  UpperLimit=HIP_MTR_MAX_TORQUE  LowerLimit=-HIP_MTR_MAX_TORQUE
      settings: AttributesFormatString=Top: %<UpperLimit>\nBottom: %<LowerLimit>
  NOT : Logic  Operator=NOT  IconShape=distinctive  AllPortsSameDT=off  OutDataTypeStr=boolean
  Ramp Rate (Units/sec) : Gain  Gain=.25
  Sagittal Motor Saturation : Saturate  UpperLimit=LEG_MTR_MAX_TORQUE  LowerLimit=-LEG_MTR_MAX_TORQUE
      settings: AttributesFormatString=Top: %<UpperLimit>\nBottom: %<LowerLimit>
  Scaling Factor : Saturate  UpperLimit=1  LowerLimit=0
  Selector : Selector  InputPortWidth=6  Indices=[1 2 4 5 6 3]
  Selector1 : Selector  InputPortWidth=6  Indices=[1 2 3 4]
  Selector2 : Selector  InputPortWidth=6  Indices=[5 6]
  Separated to Tau : Selector  InputPortWidth=6  Indices=[1 2 6 3 4 5]
  Startup Tau Ramp : Product
  Sum : Sum  Inputs=|-+
  Terminator : Terminator
  Vector Concatenate : Concatenate
  is_start_done_cmp : RelationalOperator  Operator=>  OutDataTypeStr=boolean
  tau_cmd_out [Nm] x6 : Outport  OutDataTypeStr=double  PortDimensions=6
  wires:
  NOT/1 -> Hold Start Time/Enable
  is_run_cmd/1 -> NOT/1
  Current Time/1 -> Enabled time/2, Hold Start Time/1(Time In)
  Hold Start Time/1(Time Out) -> Enabled time/1
  Enabled time/1 -> Ramp Rate (Units/sec)/1
  Ramp Rate (Units/sec)/1 -> Scaling Factor/1, Sum/2
  Scaling Factor/1 -> is_start_done_cmp/2, Startup Tau Ramp/1
  Startup Tau Ramp/1 -> tau_cmd_out [Nm] x6/1
  Selector2/1 -> Lateral Motor Saturation/1  "lateral"
  Selector1/1 -> Sagittal Motor Saturation/1  "sagittal"
  tau_cmd_in [Nm] x6/1 -> Selector/1
  Selector/1 -> Selector1/1, Selector2/1
  Sagittal Motor Saturation/1 -> Vector Concatenate/1
  Lateral Motor Saturation/1 -> Vector Concatenate/2
  Vector Concatenate/1 -> Separated to Tau/1
  Separated to Tau/1 -> Startup Tau Ramp/2
  Sum/1 -> is_start_done_cmp/1
  is_start_done_cmp/1 -> Terminator/1

== system atrias_system/Substitute Hip Positions ==
  Absolute : Inport
  Incremental : Inport  Port=2
  Mux1 : Mux  Inputs=2
  Replace Hips with Incremental : Selector  InputPortWidth=19  Indices=[1 2 3 4 5 6 7 8 18 19 11 12 13]
  Reshape : Reshape
  Substituted : Outport
  wires:
  Incremental/1 -> Mux1/2
  Absolute/1 -> Mux1/1
  Replace Hips with Incremental/1 -> Reshape/1
  Mux1/1 -> Replace Hips with Incremental/1
  Reshape/1 -> Substituted/1

== system atrias_system/Substitute Hip Velocities ==
  Absolute : Inport
  Incremental : Inport  Port=2
  Mux1 : Mux  Inputs=2
  Replace Hips with Incremental : Selector  InputPortWidth=19  Indices=[1 2 3 4 5 6 7 8 18 19 11 12 13]
  Reshape : Reshape
  Substituted : Outport
  wires:
  Reshape/1 -> Substituted/1
  Mux1/1 -> Replace Hips with Incremental/1
  Replace Hips with Incremental/1 -> Reshape/1
  Absolute/1 -> Mux1/1
  Incremental/1 -> Mux1/2

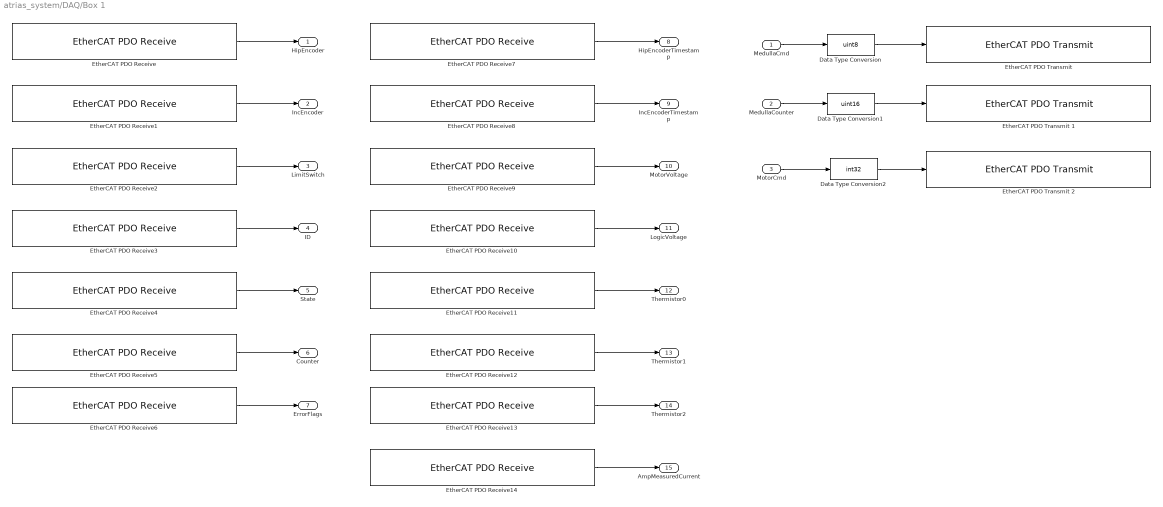
== system atrias_system/DAQ/Box 1 ==
  MedullaCmd : Inport
  MedullaCounter : Inport  Port=2
  MotorCmd : Inport  Port=3
  Data Type Conversion : DataTypeConversion  OutDataTypeStr=uint8
  Data Type Conversion1 : DataTypeConversion  OutDataTypeStr=uint16
  Data Type Conversion2 : DataTypeConversion  OutDataTypeStr=int32
  EtherCAT PDO Receive : xpcethercatlib/EtherCAT PDO Receive  Priority=2  sig_name=Box 1 (ATRIAS 2.1 Hip (Medulla 1.5)).Hip Encoder.Encoder  sig_offset=632  sig_type=uint32  type_size=32  sig_dim=1  device_id=0  sample_time=0.001000
  EtherCAT PDO Receive1 : xpcethercatlib/EtherCAT PDO Receive  Priority=2  sig_name=Box 1 (ATRIAS 2.1 Hip (Medulla 1.5)).Incremental Encoder.Incremental Encoder  sig_offset=776  sig_type=uint16  type_size=16  sig_dim=1  device_id=0  sample_time=0.001000
  EtherCAT PDO Receive10 : xpcethercatlib/EtherCAT PDO Receive  Priority=2  sig_name=Box 1 (ATRIAS 2.1 Hip (Medulla 1.5)).Power.Logic Voltage  sig_offset=696  sig_type=uint16  type_size=16  sig_dim=1  device_id=0  sample_time=0.001000
  EtherCAT PDO Receive11 : xpcethercatlib/EtherCAT PDO Receive  Priority=2  sig_name=Box 1 (ATRIAS 2.1 Hip (Medulla 1.5)).Thermistors.Thermistor 0  sig_offset=712  sig_type=uint16  type_size=16  sig_dim=1  device_id=0  sample_time=0.001000
  EtherCAT PDO Receive12 : xpcethercatlib/EtherCAT PDO Receive  Priority=2  sig_name=Box 1 (ATRIAS 2.1 Hip (Medulla 1.5)).Thermistors.Thermistor 1  sig_offset=728  sig_type=uint16  type_size=16  sig_dim=1  device_id=0  sample_time=0.001000
  EtherCAT PDO Receive13 : xpcethercatlib/EtherCAT PDO Receive  Priority=2  sig_name=Box 1 (ATRIAS 2.1 Hip (Medulla 1.5)).Thermistors.Thermistor 2  sig_offset=744  sig_type=uint16  type_size=16  sig_dim=1  device_id=0  sample_time=0.001000
  EtherCAT PDO Receive14 : xpcethercatlib/EtherCAT PDO Receive  Priority=2  sig_name=Box 1 (ATRIAS 2.1 Hip (Medulla 1.5)).Measured Current.Amp Measured Current  sig_offset=760  sig_type=int16  type_size=16  sig_dim=1  device_id=0  sample_time=0.001000
  EtherCAT PDO Receive2 : xpcethercatlib/EtherCAT PDO Receive  Priority=2  sig_name=Box 1 (ATRIAS 2.1 Hip (Medulla 1.5)).uController Status.Limit Switch  sig_offset=624  sig_type=uint8  type_size=8  sig_dim=1  device_id=0  sample_time=0.001000
  EtherCAT PDO Receive3 : xpcethercatlib/EtherCAT PDO Receive  Priority=2  sig_name=Box 1 (ATRIAS 2.1 Hip (Medulla 1.5)).uController Status.ID  sig_offset=592  sig_type=uint8  type_size=8  sig_dim=1  device_id=0  sample_time=0.001000
  EtherCAT PDO Receive4 : xpcethercatlib/EtherCAT PDO Receive  Priority=2  sig_name=Box 1 (ATRIAS 2.1 Hip (Medulla 1.5)).uController Status.State  sig_offset=600  sig_type=uint8  type_size=8  sig_dim=1  device_id=0  sample_time=0.001000
  EtherCAT PDO Receive5 : xpcethercatlib/EtherCAT PDO Receive  Priority=2  sig_name=Box 1 (ATRIAS 2.1 Hip (Medulla 1.5)).uController Status.Counter  sig_offset=608  sig_type=uint8  type_size=8  sig_dim=1  device_id=0  sample_time=0.001000
  EtherCAT PDO Receive6 : xpcethercatlib/EtherCAT PDO Receive  Priority=2  sig_name=Box 1 (ATRIAS 2.1 Hip (Medulla 1.5)).uController Status.Error Flags  sig_offset=616  sig_type=uint8  type_size=8  sig_dim=1  device_id=0  sample_time=0.001000
  EtherCAT PDO Receive7 : xpcethercatlib/EtherCAT PDO Receive  Priority=2  sig_name=Box 1 (ATRIAS 2.1 Hip (Medulla 1.5)).Hip Encoder.Timestamp  sig_offset=664  sig_type=uint16  type_size=16  sig_dim=1  device_id=0  sample_time=0.001000
  EtherCAT PDO Receive8 : xpcethercatlib/EtherCAT PDO Receive  Priority=2  sig_name=Box 1 (ATRIAS 2.1 Hip (Medulla 1.5)).Incremental Encoder.Incremental Encoder Timestamp  sig_offset=792  sig_type=uint16  type_size=16  sig_dim=1  device_id=0  sample_time=0.001000
  EtherCAT PDO Receive9 : xpcethercatlib/EtherCAT PDO Receive  Priority=2  sig_name=Box 1 (ATRIAS 2.1 Hip (Medulla 1.5)).Power.Motor Voltage  sig_offset=680  sig_type=uint16  type_size=16  sig_dim=1  device_id=0  sample_time=0.001000
  "EtherCAT PDO Transmit " : xpcethercatlib/EtherCAT PDO Transmit   Priority=3  sig_name=Box 1 (ATRIAS 2.1 Hip (Medulla 1.5)).uControllerInput.Command  sig_offset=592  sig_type=uint8  type_size=8  sig_dim=1  device_id=0  sample_time=0.001000
  EtherCAT PDO Transmit 1 : xpcethercatlib/EtherCAT PDO Transmit   Priority=3  sig_name=Box 1 (ATRIAS 2.1 Hip (Medulla 1.5)).uControllerInput.Counter  sig_offset=600  sig_type=uint16  type_size=16  sig_dim=1  device_id=0  sample_time=0.001000
  EtherCAT PDO Transmit 2 : xpcethercatlib/EtherCAT PDO Transmit   Priority=3  sig_name=Box 1 (ATRIAS 2.1 Hip (Medulla 1.5)).uControllerInput.Motor Current  sig_offset=616  sig_type=int32  type_size=32  sig_dim=1  device_id=0  sample_time=0.001000
  HipEncoder : Outport
  IncEncoder : Outport  Port=2
  LimitSwitch : Outport  Port=3
  ID : Outport  Port=4
  State : Outport  Port=5
  Counter : Outport  Port=6
  ErrorFlags : Outport  Port=7
  HipEncoderTimestamp : Outport  Port=8
  IncEncoderTimestamp : Outport  Port=9
  MotorVoltage : Outport  Port=10
  LogicVoltage : Outport  Port=11
  Thermistor0 : Outport  Port=12
  Thermistor1 : Outport  Port=13
  Thermistor2 : Outport  Port=14
  AmpMeasuredCurrent : Outport  Port=15
  wires:
  Data Type Conversion/1 -> "EtherCAT PDO Transmit "/1
  Data Type Conversion1/1 -> EtherCAT PDO Transmit 1/1
  Data Type Conversion2/1 -> EtherCAT PDO Transmit 2/1
  MedullaCmd/1 -> Data Type Conversion/1
  MedullaCounter/1 -> Data Type Conversion1/1
  MotorCmd/1 -> Data Type Conversion2/1
  EtherCAT PDO Receive8/1 -> IncEncoderTimestamp/1
  EtherCAT PDO Receive/1 -> HipEncoder/1
  EtherCAT PDO Receive7/1 -> HipEncoderTimestamp/1
  EtherCAT PDO Receive1/1 -> IncEncoder/1
  EtherCAT PDO Receive5/1 -> Counter/1
  EtherCAT PDO Receive3/1 -> ID/1
  EtherCAT PDO Receive2/1 -> LimitSwitch/1
  EtherCAT PDO Receive4/1 -> State/1
  EtherCAT PDO Receive6/1 -> ErrorFlags/1
  EtherCAT PDO Receive10/1 -> LogicVoltage/1
  EtherCAT PDO Receive9/1 -> MotorVoltage/1
  EtherCAT PDO Receive11/1 -> Thermistor0/1
  EtherCAT PDO Receive12/1 -> Thermistor1/1
  EtherCAT PDO Receive13/1 -> Thermistor2/1
  EtherCAT PDO Receive14/1 -> AmpMeasuredCurrent/1
